simulink model "fw_att_control"  (R2021a)
settings: Solver=FixedStepAuto  StartTime=0.0  StopTime=10.0  RelTol=1e-3
undefined symbols (not defined in the file): DiscIntNeverNeededParam, FW_ACRO_X_MAX, FW_ACRO_Y_MAX, FW_ACRO_Z_MAX, FW_AIRSPD_MAX, FW_AIRSPD_STALL, FW_AIRSPD_TRIM, FW_BAT_SCALE_EN, FW_DTRIM_P_FLPS, FW_DTRIM_P_VMAX, FW_DTRIM_P_VMIN, FW_DTRIM_R_FLPS, FW_DTRIM_R_VMAX, FW_DTRIM_R_VMIN, FW_DTRIM_Y_VMAX, FW_DTRIM_Y_VMIN, FW_FLAPERON_SCL, FW_FLAPS_LND_SCL, FW_FLAPS_SCL, FW_FLAPS_TO_SCL, FW_MAN_P_MAX, FW_MAN_P_SC, FW_MAN_R_MAX, FW_MAN_R_SC, FW_MAN_Y_SC, FW_P_TC, FW_PR_IMAX, FW_PR_P, FW_PSP_OFF, FW_R_TC, FW_RLL_TO_YAW_FF, FW_RR_FF, FW_W_EN, FW_W_RMAX, FW_WR_FF, FW_WR_P, FW_Y_TC, FW_YR_FF, FW_YR_P, magnitude, PX4_VEHICLE_ATTITUDE_SETPOINT, PX4_VEHICLE_STATUS, TRIM_PITCH, TRIM_ROLL, TRIM_YAW
libraries: simulink x10, aerolibconvert2 x5, sharedtransform x2
(part 2 of 2)

== system fw_att_control/Rate Control/Wheel Rate Control/积分项 ==
  yaw_rate_error : Inport
  Abs : Abs
  Bus Selector : BusSelector  OutputSignals=lock_integrator
  Bus Selector1 : BusSelector  OutputSignals=reset_yaw_i
  Compare To Constant : simulink/Logic and Bit Operations/Compare To Constant  relop=>  const=1  OutDataTypeStr=boolean
  Constant : Constant  Value=0
  Discrete-Time Integrator1 : DiscreteIntegrator  gainval=FW_RR_I  ExternalReset=level  SampleTime=-1  LimitOutput=on  UpperSaturationLimit=FW_PR_IMAX  LowerSaturationLimit=-FW_PR_IMAX  ICPrevOutput=DiscIntNeverNeededParam  ICPrevScaledInput=DiscIntNeverNeededParam
  Math Function2 : Math  Operator=magnitude^2  SaturateOnIntegerOverflow=on
  NOT : Logic  Operator=NOT  IconShape=distinctive  AllPortsSameDT=off  OutDataTypeStr=boolean
  Product1 : Product  Inputs=3
  Switch : Switch  Criteria=u2 > Threshold
  out : Outport
  wires:
  yaw_rate_error/1 -> Product1/2
  Math Function2/1 -> Product1/3
  NOT/1 -> Product1/1
  Discrete-Time Integrator1/1 -> out/1
  [gspd_scaler] -> Math Function2/1
  [integrator_flag] -> Bus Selector/1
  Bus Selector/1 -> NOT/1  "<lock_integrator>"
  [integrator_flag] -> Bus Selector1/1
  Bus Selector1/1 -> Discrete-Time Integrator1/2  "<reset_yaw_i>"
  Abs/1 -> Compare To Constant/1
  Compare To Constant/1 -> Switch/2
  [yaw_wheel_output] -> Abs/1
  Product1/1 -> Switch/3  "yaw_id"
  Constant/1 -> Switch/1
  Switch/1 -> Discrete-Time Integrator1/1

== system fw_att_control/Rate Control/Yaw Rate Control/前馈项 ==
  yaw_bodyrate_sp : Inport
  Gain : Gain  Gain=FW_YR_FF
  Product : Product
  out : Outport
  wires:
  [airspd_scaler] -> Product/1
  Gain/1 -> Product/2
  Product/1 -> out/1
  yaw_bodyrate_sp/1 -> Gain/1

== system fw_att_control/Rate Control/Yaw Rate Control/比例项 ==
  yaw_rate_error : Inport
  Gain2 : Gain  Gain=FW_YR_P
  Math Function : Math  Operator=magnitude^2  SaturateOnIntegerOverflow=on
  Product : Product
  out : Outport
  wires:
  [airspd_scaler] -> Math Function/1
  Product/1 -> out/1
  Gain2/1 -> Product/2
  Math Function/1 -> Product/1
  yaw_rate_error/1 -> Gain2/1

== system fw_att_control/Rate Control/Yaw Rate Control/积分项 ==
  yaw_rate_error : Inport
  Abs : Abs
  Bus Selector : BusSelector  OutputSignals=lock_integrator
  Bus Selector1 : BusSelector  OutputSignals=reset_yaw_i
  Compare To Constant : simulink/Logic and Bit Operations/Compare To Constant  relop=>  const=1  OutDataTypeStr=boolean
  Constant : Constant  Value=0  OutDataTypeStr=single
  Discrete-Time Integrator1 : DiscreteIntegrator  gainval=FW_RR_I  ExternalReset=level  SampleTime=-1  LimitOutput=on  UpperSaturationLimit=FW_PR_IMAX  LowerSaturationLimit=-FW_PR_IMAX  ICPrevOutput=DiscIntNeverNeededParam  ICPrevScaledInput=DiscIntNeverNeededParam
  Math Function2 : Math  Operator=magnitude^2  SaturateOnIntegerOverflow=on
  NOT : Logic  Operator=NOT  IconShape=distinctive  AllPortsSameDT=off  OutDataTypeStr=boolean
  Product1 : Product  Inputs=3
  Switch : Switch  Criteria=u2 > Threshold
  out : Outport
  wires:
  [airspd_scaler] -> Math Function2/1
  Discrete-Time Integrator1/1 -> out/1
  NOT/1 -> Product1/1
  Math Function2/1 -> Product1/3
  yaw_rate_error/1 -> Product1/2
  [integrator_flag] -> Bus Selector/1
  Bus Selector/1 -> NOT/1  "<lock_integrator>"
  [integrator_flag] -> Bus Selector1/1
  Bus Selector1/1 -> Discrete-Time Integrator1/2  "<reset_yaw_i>"
  [yaw_last_output] -> Abs/1
  Abs/1 -> Compare To Constant/1
  Compare To Constant/1 -> Switch/2
  Constant/1 -> Switch/1
  Product1/1 -> Switch/3  "yaw_id"
  Switch/1 -> Discrete-Time Integrator1/1

== system fw_att_control/Fix Control Yaw/Flaps Control/If Action Subsystem3/If Action Subsystem ==
  Action Port : ActionPort  ActionPortLabel=case [ 0 ]:
  Constant : Constant  Value=0  OutDataTypeStr=single
  flap_control : Outport
  wires:
  Constant/1 -> flap_control/1

== system fw_att_control/Fix Control Yaw/Flaps Control/If Action Subsystem3/If Action Subsystem1 ==
  Action Port : ActionPort  ActionPortLabel=case [ 1 ]:
  Constant1 : Constant  Value=FW_FLAPS_SCL  OutDataTypeStr=single
  Constant2 : Constant  Value=FW_FLAPS_LND_SCL  OutDataTypeStr=single
  Product : Product
  flap_control : Outport
  wires:
  Product/1 -> flap_control/1
  Constant1/1 -> Product/1
  Constant2/1 -> Product/2

== system fw_att_control/Fix Control Yaw/Flaps Control/If Action Subsystem3/If Action Subsystem2 ==
  Action Port : ActionPort  ActionPortLabel=case [ 2 ]:
  Constant1 : Constant  Value=FW_FLAPS_SCL  OutDataTypeStr=single
  Constant2 : Constant  Value=FW_FLAPS_TO_SCL  OutDataTypeStr=single
  Product : Product
  flap_control : Outport
  wires:
  Constant2/1 -> Product/2
  Product/1 -> flap_control/1
  Constant1/1 -> Product/1

== stateflow chart fw_att_control/Chart ==
  state auto_mode
    en,du:
    auto_mode = 2;
    rate_mode = 0;
  state att
    en,du:
    auto_mode = 1;
    rate_mode =1;
  state rate
    en,du:
    auto_mode = 1;
    rate_mode = 2;
  state dir
    en,du:
    auto_mode = 1;
    rate_mode = 0;
  (default) -> (junction 141) : {auto_mode = 0;
      | rate_mode = 0;}
  (junction 141) -> auto_mode [order 2]
  (junction 141) -> (junction 180) [order 1] : [mode.flag_control_manual_enabled]
  (junction 180) -> dir [order 3] : [~mode.flag_control_climb_rate_enabled]
  (junction 180) -> rate [order 2] : [~mode.flag_control_climb_rate_enabled && ...
      | mode.flag_control_rates_enabled]
  (junction 180) -> att [order 1] : [~mode.flag_control_climb_rate_enabled && ...
      | mode.flag_control_attitude_enabled]
  data: mode input; auto_mode output; rate_mode output
